simulink model "scheduling"  (R2018a)
settings: Solver=VariableStepAuto  StartTime=0.0  StopTime=10.0  RelTol=1e-3
undefined symbols (not defined in the file or in its folder): C1, C2
libraries: truetime x4, dspsigops x2
settings Model: Creator=pschalkwijk  LastModifiedBy=pschalkwijk

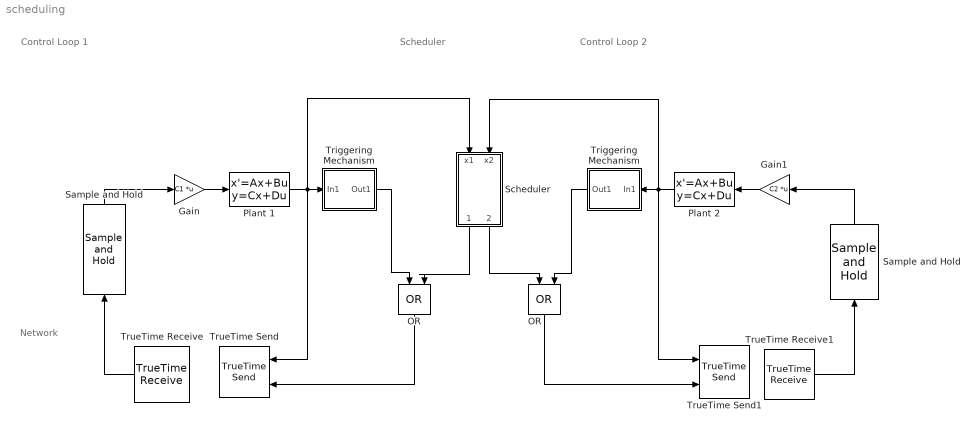
== system scheduling ==
  note: Scheduler
  note: Control Loop 1
  note: Network
  note: Control Loop 2
  Gain : Gain  Gain=C1  Multiplication=Matrix(K*u)
  Gain1 : Gain  Gain=C2  Multiplication=Matrix(K*u)
  "OR " : Logic  Operator=OR  IconShape=distinctive  AllPortsSameDT=off  OutDataTypeStr=boolean
  "OR  " : Logic  Operator=OR  IconShape=distinctive  AllPortsSameDT=off  OutDataTypeStr=boolean
  "Plant 1 " : StateSpace  InitialCondition=0
  "Plant 2 " : StateSpace  InitialCondition=0
  Sample and Hold : dspsigops/Sample and Hold  trig=Rising edge  initCond=0  latchinput=on
  "Sample and Hold " : dspsigops/Sample and Hold  trig=Rising edge  initCond=0  latchinput=on
  Scheduler : Subsystem
  "Triggering Mechanism " : Subsystem
  "Triggering Mechanism " : Subsystem
  TrueTime Receive : truetime/TrueTime Receive  nwnbr=1  receiver=1  outdim=1  triggeroutput=off  senderoutput=off  lengthoutput=off  priorityoutput=off  timestampoutput=off  signalpoweroutput=off  msgIDoutput=off
  TrueTime Receive1 : truetime/TrueTime Receive  nwnbr=1  receiver=2  outdim=1  triggeroutput=off  senderoutput=off  lengthoutput=off  priorityoutput=off  timestampoutput=off  signalpoweroutput=off  msgIDoutput=off
  TrueTime Send : truetime/TrueTime Send  trigger=falling  nwnbr=1  sender=1  indim=1  recsource=internal  receiver=1  lengthsource=internal  length=1000  priosource=internal  prio=1  msgIDsource=internal  msgID=0  dynamicSegment=dynamic
  TrueTime Send1 : truetime/TrueTime Send  trigger=falling  nwnbr=1  sender=2  indim=1  recsource=internal  receiver=2  lengthsource=internal  length=1000  priosource=internal  prio=1  msgIDsource=internal  msgID=0  dynamicSegment=dynamic
  wires:
  "Plant 1 "/1 -> TrueTime Send/1, "Triggering Mechanism "/1(In1), Scheduler/1(x1)
  Gain/1 -> "Plant 1 "/1
  Sample and Hold/1 -> Gain/1
  TrueTime Receive/1 -> Sample and Hold/1
  "Plant 2 "/1 -> Scheduler/2(x2), TrueTime Send1/1, "Triggering Mechanism "/1(In1)
  Gain1/1 -> "Plant 2 "/1
  TrueTime Receive1/1 -> "Sample and Hold "/1
  "OR  "/1 -> TrueTime Send/2
  "OR "/1 -> TrueTime Send1/2
  "Triggering Mechanism "/1(Out1) -> "OR "/2
  Scheduler/1(Trig1) -> "OR  "/2
  Scheduler/2(Trig2) -> "OR "/1
  "Sample and Hold "/1 -> Gain1/1
  "Triggering Mechanism "/1(Out1) -> "OR  "/1

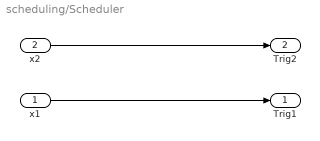
== system scheduling/Scheduler ==
  x1 : Inport
  x2 : Inport  Port=2
  Trig1 : Outport
  Trig2 : Outport  Port=2
  wires:
  x1/1 -> Trig1/1
  x2/1 -> Trig2/1

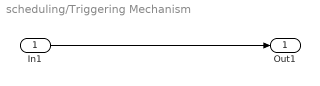
== system scheduling/Triggering Mechanism  ==
  In1 : Inport
  Out1 : Outport
  wires:
  In1/1 -> Out1/1

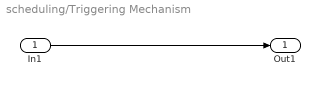
== system scheduling/Triggering Mechanism  ==
  In1 : Inport
  Out1 : Outport
  wires:
  In1/1 -> Out1/1
